simulink model "derivativecalculater"  (R2016b)
settings: Solver=VariableStepAuto  StartTime=0.0  StopTime=10.0  RelTol=1e-3
settings Model: DataDictionary=DataDictionary.sldd  Creator=Taeke  LastModifiedBy=march

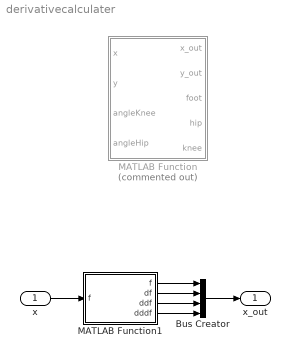
== system derivativecalculater ==
  x : Inport  PortDimensions=numberSamplePoints
  Bus Creator : BusCreator  Inputs=4
  MATLAB Function : MATLAB Function  Commented=on  TreatAsAtomicUnit=on
  MATLAB Function1 : MATLAB Function  TreatAsAtomicUnit=on
  x_out : Outport
  wires:
  MATLAB Function1/1(f) -> Bus Creator/1
  MATLAB Function1/3(ddf) -> Bus Creator/3
  MATLAB Function1/2(df) -> Bus Creator/2
  MATLAB Function1/4(dddf) -> Bus Creator/4
  x/1 -> MATLAB Function1/1("f ")
  Bus Creator/1 -> x_out/1

== matlab function derivativecalculater/MATLAB Function ==
  data: x_out output; y_out output; x input; foot output; y input; hip output; knee output; angleKnee input; angleHip input
function [x_out, y_out, foot, hip, knee] = fcn(x, y, angleKnee, angleHip)
t = 0.1*4/100; %[s]
[dx, dxx, ddx] = derivatives(x,t);
x_out = [x, dx, dxx, ddx];

[dx, dxx, ddx] = derivatives(y,t);
y_out = [y, dx, dxx, ddx];

foot_position = sqrt(x.^2+y.^2);
[dx, dxx, ddx] = derivatives(foot_position,t);
foot = [ foot_position,dx, dxx, ddx];

[dx, dxx, ddx] = derivatives(angleKnee, t);
knee = [angleKnee dx, dxx, ddx];

[dx, dxx, ddx] = derivatives(angleHip, t);
hip = [angleHip, dx, dxx, ddx];

end

== matlab function derivativecalculater/MATLAB Function1 ==
  data: f input; f output; df output; ddf output; dddf output

function [f, df, ddf, dddf] = fcn(f)
t = 0.1*4/100; %[s]
[df, ddf, dddf] = derivatives(f,t);
end
